simulink model "ej2b_sin_controlador"  (R2021a)
settings: Solver=VariableStepAuto  StartTime=0.0  StopTime=2000  RelTol=1e-3
values from neighbouring files (symbols this model uses):
  h0 = h0_valores(i)    [EJ1.m]    (also in EJ2.m = 0.45; ej1b.m = 0.45; ej1e.m; ej2a.m = 0.45)
  u0 = Q_i / (A_o * sqrt(2 * g * h0))    [EJ1.m]    (also in EJ2.m; ej1b.m; ej1e.m; ej2a.m)
libraries: cstblocks x3
settings Model: Creator=franc  LastModifiedBy=facun

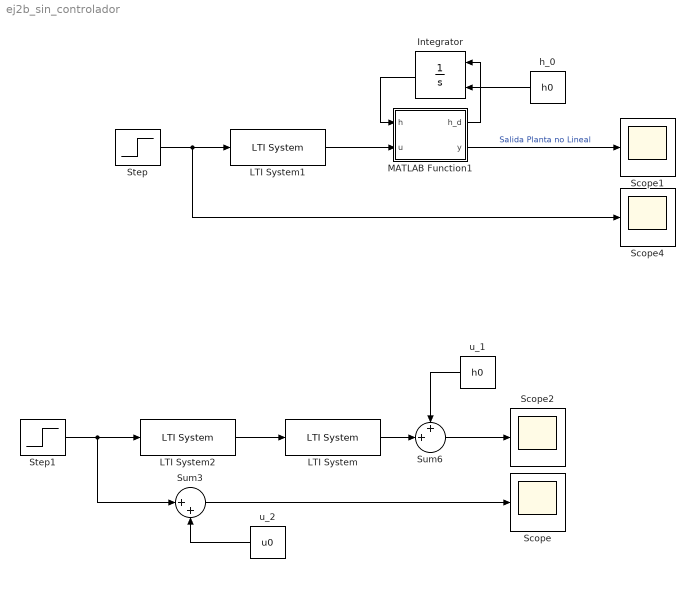
== system ej2b_sin_controlador ==
  Integrator : Integrator  InitialConditionSource=external
  LTI System : cstblocks/LTI System  sys=Pmp  IC=[]
  LTI System1 : cstblocks/LTI System  sys=1  IC=[]
  LTI System2 : cstblocks/LTI System  sys=1  IC=[]
  MATLAB Function1 : MATLAB Function  TreatAsAtomicUnit=on
  Scope{,1..2,4} (4 alike) : Scope
  Step : Step  Time=100  Before=u0  After=1.1*u0  SampleTime=0
  Step1 : Step  Time=100  After=0.05  SampleTime=0
  Sum3 : Sum  Inputs=|++
  Sum6 : Sum  Inputs=++|
  h_0 : Constant  Value=h0
  u_1 : Constant  Value=h0
  u_2 : Constant  Value=u0
  wires:
  MATLAB Function1/2(y) -> Scope1/1  "Salida Planta no Lineal"
  MATLAB Function1/1(h_d) -> Integrator/1
  h_0/1 -> Integrator/2
  Step1/1 -> LTI System2/1, Sum3/1
  Step/1 -> Scope4/1, LTI System1/1
  LTI System1/1 -> MATLAB Function1/2(u)
  u_1/1 -> Sum6/1
  LTI System2/1 -> LTI System/1
  Sum6/1 -> Scope2/1
  LTI System/1 -> Sum6/2
  u_2/1 -> Sum3/2
  Integrator/1 -> MATLAB Function1/1(h)
  Sum3/1 -> Scope/1

== matlab function ej2b_sin_controlador/MATLAB Function1 ==
  data: h input; h_d output; u input; y output
function [h_d, y] = fcn(h, u)
    g = 9.8;        %En metros sobre segundo cuadrado
    H = 0.9;        %En metros
    L_s = 0.4;      %En metros
    L_i = 0.1;      %En metros
    d2 = 10.65e-3;
    Q_i = 0.0001333; %Metros cubicos por segundo 
    A_o = pi * (d2 / 2)^2;
    h_d = (H^2 * (Q_i - A_o * sqrt(2*g*h)*u))/(h^2*(L_s-L_i)^2 + 2*h*L_i*(L_s-L_i)*H+L_i^2*H^2);
    y = h;
end
